simulink subsystem "Sub_Controller"  (R2020a)
settings: Solver=VariableStepAuto  StartTime=0.0  StopTime=10.0  RelTol=1e-3
libraries: mpclib x1
settings Model: Creator=Lamarre  LastModifiedBy=Lamarre

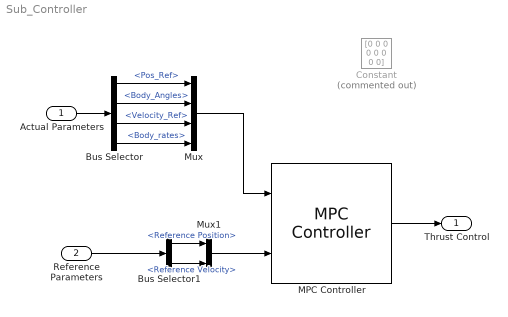
== system Sub_Controller ==
  Actual Parameters : Inport
  Reference Parameters : Inport  Port=2
  Bus Selector : BusSelector  OutputSignals=Pos_Ref,Body_Angles,Velocity_Ref,Body_rates
  Bus Selector1 : BusSelector  OutputSignals=Reference Position,Reference Velocity
  Constant : Constant  Commented=on  Value=[0 0 0 0 0 0 0 0]
  MPC Controller : mpclib/MPC Controller  SCDEnableBlockLinearizationSpecification=on  is_multiple=0  enable_value=0  return_u0=off  updateMPCinCallerWorkspace=on  md_inport=off  mv_inport=off  uref_inport=off  return_cost=off  return_mvseq=off  return_qpstatus=off  return_xseq=off  return_state=off  return_ovseq=off  state_inport=off  umin_inport=off  umax_inport=off  ymin_inport=off  ymax_inport=off  cc_inport=off  ywt_inport=off  uwt_inport=off  duwt_inport=off  rhoeps_inport=off  pm_inport=off  MaximumP=10  HorizonChoice=FixedHorizon  n_ts=0.1  n_p=10  n_mv=8  n_md=1  n_ud=0  n_mo=12  n_uo=0  BlockDataType=double  SampleTimeInherited=off  switch_inport=off
  Mux : Mux
  Mux1 : Mux  Inputs=2
  Thrust Control : Outport  VectorParamsAs1DForOutWhenUnconnected=off
  wires:
  Bus Selector1/1 -> Mux1/1  "<Reference Position>"
  Mux1/1 -> MPC Controller/2
  Bus Selector/3 -> Mux/3  "<Velocity_Ref>"
  Bus Selector/2 -> Mux/2  "<Body_Angles>"
  Actual Parameters/1 -> Bus Selector/1
  Mux/1 -> MPC Controller/1
  MPC Controller/1 -> Thrust Control/1
  Reference Parameters/1 -> Bus Selector1/1
  Bus Selector/4 -> Mux/4  "<Body_rates>"
  Bus Selector/1 -> Mux/1  "<Pos_Ref>"
  Bus Selector1/2 -> Mux1/2  "<Reference Velocity>"
